simulink model "Calc1"  (R2018b)
settings: Solver=FixedStepDiscrete  StartTime=0.0  StopTime=10.0  RelTol=1e-3
settings Model: Creator=Mostafa  LastModifiedBy=Mostafa
settings ConfigSet: Description=Mostafa Hany Imam
settings OptimizationCC: DefaultParameterBehavior=Inlined  EnhancedBackFolding=on  PassReuseOutputArgsAs=Individual arguments  OptimizeBlockOrder=speed  DifferentSizesBufferReuse=on  OptimizationCustomize=off
settings DebuggingCC: UnderspecifiedInitializationDetection=Classic  MergeDetectMultiDrivingBlocksExec=none  ParameterTunabilityLossMsg=error
settings ModelReferenceCC: PropagateSignalLabelsOutOfModel=off
settings SFSimCC: MATLABDynamicMemAlloc=off
settings RTWCC: SystemTargetFile=ert.tlc  GenCodeOnly=on  TemplateMakefile=ert_default_tmf  GenerateReport=on  IncludeHyperlinkInReport=on  LaunchReport=on  GenerateTraceInfo=on  GenerateTraceReport=on  GenerateTraceReportSl=on  GenerateTraceReportSf=on  GenerateTraceReportEml=on
settings CodeAppCC: ForceParamTrailComments=on  IgnoreCustomStorageClasses=off  OperatorAnnotations=on  SimulinkDataObjDesc=on  SFDataObjDesc=on  InsertBlockDesc=on
settings ERTTargetCC: TargetLangStandard=C99 (ISO)  GenerateSampleERTMain=on  InlinedParameterPlacement=NonHierarchical  ERTCustomFileTemplate=example_file_process.tlc

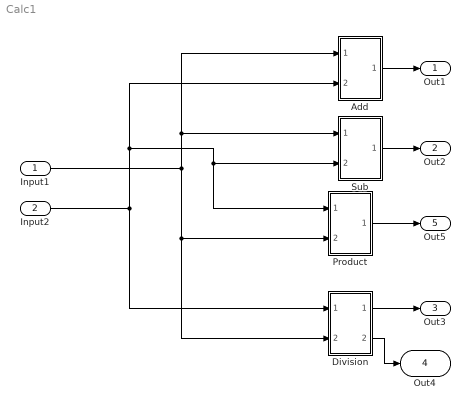
== system Calc1 ==
  "Input1 " : Inport
  "Input2 " : Inport  Port=2
  Add : Subsystem
  "Division " : Subsystem
  "Product " : Subsystem
  "Sub " : Subsystem
  Out1 : Outport  SignalName=Add
  Out2 : Outport  Port=2  SignalName=Subtract
  Out3 : Outport  Port=3  SignalName=Divide
  Out4 : Outport  Port=4  SignalName=ErrorFlag
  Out5 : Outport  Port=5  SignalName=Product
  wires:
  "Input1 "/1 -> Add/1(In1), "Sub "/1(In1), "Division "/2(In2), "Product "/2(In2)
  "Input2 "/1 -> Add/2(In2), "Product "/1(In1), "Sub "/2(In2), "Division "/1(In1)
  Add/1(Out1) -> Out1/1
  "Sub "/1(Out2) -> Out2/1
  "Product "/1(Out5) -> Out5/1
  "Division "/1(Out3) -> Out3/1
  "Division "/2(Out4) -> Out4/1

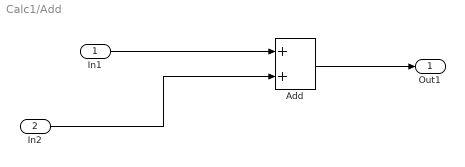
== system Calc1/Add ==
  In1 : Inport
  In2 : Inport  Port=2
  Add : Sum
  Out1 : Outport
  wires:
  Add/1 -> Out1/1
  In2/1 -> Add/2
  In1/1 -> Add/1

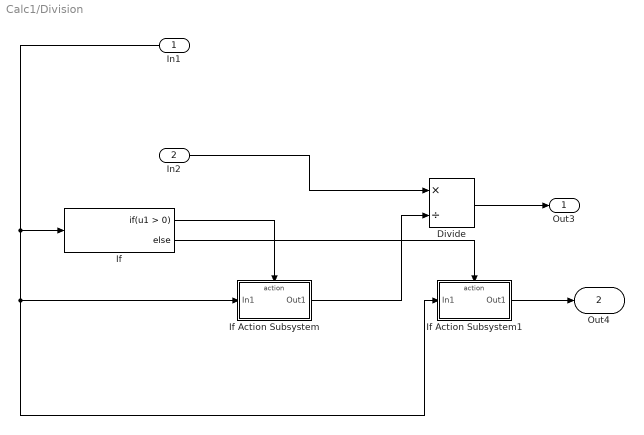
== system Calc1/Division  ==
  In1 : Inport
  In2 : Inport  Port=2
  Divide : Product  Inputs=*/
  If : If
  If Action Subsystem : Subsystem  TreatAsAtomicUnit=on
  If Action Subsystem1 : Subsystem  TreatAsAtomicUnit=on
  Out3 : Outport
  Out4 : Outport  Port=2
  wires:
  In1/1 -> If Action Subsystem1/1(In1), If Action Subsystem/1(In1), If/1
  Divide/1 -> Out3/1
  If/2 -> If Action Subsystem1/Action
  If Action Subsystem/1(Out1) -> Divide/2
  If Action Subsystem1/1(Out1) -> Out4/1
  If/1 -> If Action Subsystem/Action
  In2/1 -> Divide/1

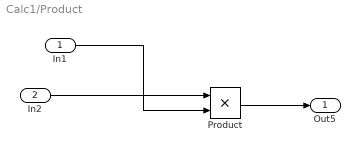
== system Calc1/Product  ==
  In1 : Inport
  In2 : Inport  Port=2
  Product : Product
  Out5 : Outport
  wires:
  Product/1 -> Out5/1
  In1/1 -> Product/2
  In2/1 -> Product/1

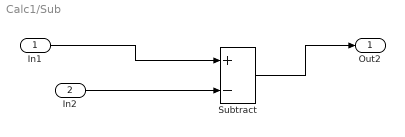
== system Calc1/Sub  ==
  In1 : Inport
  In2 : Inport  Port=2
  Subtract : Sum  Inputs=+-
  Out2 : Outport
  wires:
  Subtract/1 -> Out2/1
  In1/1 -> Subtract/1
  In2/1 -> Subtract/2

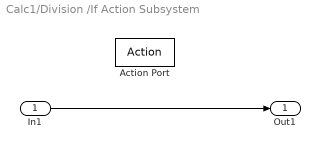
== system Calc1/Division /If Action Subsystem ==
  In1 : Inport
  Action Port : ActionPort  ActionType=then
  Out1 : Outport
  wires:
  In1/1 -> Out1/1

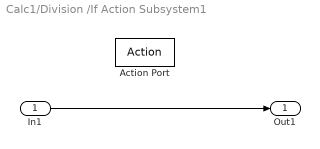
== system Calc1/Division /If Action Subsystem1 ==
  In1 : Inport
  Action Port : ActionPort  ActionType=else
  Out1 : Outport
  wires:
  In1/1 -> Out1/1
